simulink model "hpipm_simulink_getting_started"  (R2017b)
settings: Solver=VariableStepAuto  StartTime=0.0  StopTime=50.0  RelTol=1e-3
values from neighbouring files (symbols this model uses):
  N = dim.get('N')    [load_parameters.m]
  NU = dim.get('nu', 0)    [load_parameters.m]
  NX = dim.get('nx', 0)    [load_parameters.m]
settings Model: Creator=andrea  LastModifiedBy=andrea

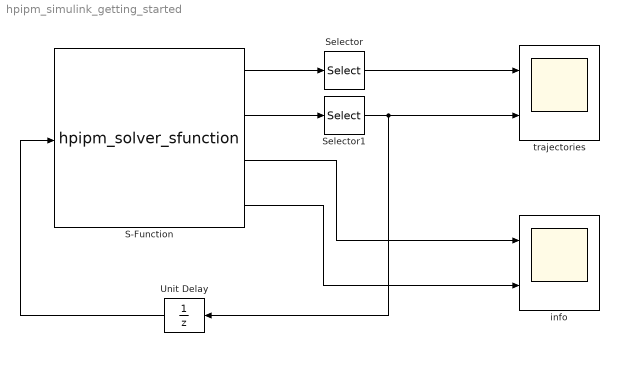
== system hpipm_simulink_getting_started ==
  S-Function : S-Function  FunctionName=hpipm_solver_sfunction  SFunctionDeploymentMode=off  EnableBusSupport=off
  Selector : Selector  InputPortWidth=NU*N  IndexOptions=Index vector (dialog)  Indices=1:NU  OutputSizes=1
  Selector1 : Selector  InputPortWidth=NX*(N+1)  IndexOptions=Index vector (dialog)  Indices=(NX+1):(2*NX)  OutputSizes=1
  Unit Delay : UnitDelay  InitialCondition=[3.5 3.5 0 0 0 0 0 0];  SampleTime=0.5
  info : Scope  NumInputPorts=2
  trajectories : Scope  NumInputPorts=2
  wires:
  S-Function/2 -> Selector1/1
  Unit Delay/1 -> S-Function/1
  S-Function/1 -> Selector/1
  Selector/1 -> trajectories/1
  Selector1/1 -> Unit Delay/1, trajectories/2
  S-Function/3 -> info/1
  S-Function/4 -> info/2
